simulink model "linearModelOpenLoop"  (Simulink 7.9)
settings: Solver=ode45  StartTime=0.0  StopTime=1  RelTol=1e-3
values from neighbouring files (symbols this model uses):
  K = lqr(A,B,Q,R)    [LQR.m]    (also in bestQ.m = setK_lqr(Q_i); graficosPenduloReal.m = setK_lqr(Q_optimo))
settings Model: Creator=root  LastModifiedBy=root

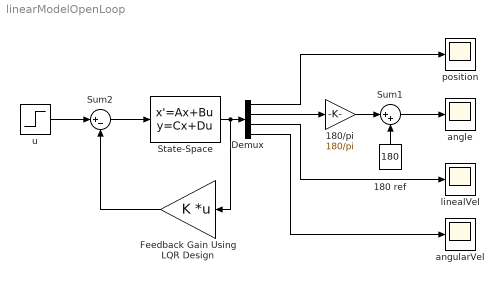
== system linearModelOpenLoop ==
  180 ref : Constant  Value=180  VectorParams1D=off
  180/pi : Gain  Gain=180/pi
  Demux : Demux
  Feedback Gain Using LQR Design : Gain  Gain=K  Multiplication=Matrix(K*u) (u vector)
  State-Space : StateSpace  A="[0 0 1 0; 0 0 0 1; 0 0.5401 -0.7235 0; 0  14.955 -0.9854 0]"  B="[0  ;0 ;2.2747 ;3.0978]"  C=eye(4)  D=[0;0;0;0]  X0=[ 0 ; -10*pi/180; 0; 0 ]
  Sum1 : Sum  Inputs=|++
  Sum2 : Sum  Inputs=|+-
  angle : Scope
      settings: TimeRange=0.35  YMin=88.25  YMax=91.75  SaveName=thetaLineal
  angularVel : Scope
      settings: SaveName=angularVelLineal
  linealVel : Scope
      settings: SaveName=linealVelLineal
  position : Scope
      settings: SaveName=positionLineal
  u : Step  Time=0  After=0  SampleTime=0
  wires:
  State-Space/1 -> Demux/1, Feedback Gain Using LQR Design/1
  Demux/1 -> position/1
  Demux/2 -> 180/pi/1
  Demux/4 -> angularVel/1
  180/pi/1 -> Sum1/1
  180 ref/1 -> Sum1/2
  Sum1/1 -> angle/1
  Demux/3 -> linealVel/1
  u/1 -> Sum2/1
  Sum2/1 -> State-Space/1
  Feedback Gain Using LQR Design/1 -> Sum2/2
